simulink model "alt_dspbuilder_internal_ReadFIFO"  (Simulink 6.3)
settings: Solver=ode45  StartTime=0.0  StopTime=10.0  RelTol=1e-3
InitFcn:
  | %% DSPBuilder Start
  | alt_dspbuilder_update_model(bdroot)
  | %% DSPBuilder End
libraries: allblocks_alteradspbuilder2 x6
settings Model: Creator=cpurcell  LastModifiedBy=cpurcell
settings DebuggingCC: AlgebraicLoopMsg=none  MultiTaskCondExecSysMsg=none  StrictBusMsg=Warning
settings RTWCC: IncludeERTFirstTime=on
settings CodeAppCC: CustomSymbolStrType=$N$R$M

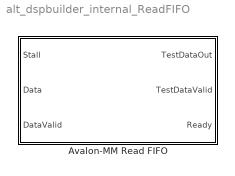
== system alt_dspbuilder_internal_ReadFIFO ==
  Avalon-MM Read FIFO : Subsystem  mask(Avalon-MM Read FIFO AlteraBlockSet){sgn=Signed Integer, bwl=8, bwr=3, depth=11, burst=0}
      mask prompts: sgn "Data Type"; bwl "[number of bits].[]"; bwr "[].[number of bits]"; depth "FIFO Depth"; burst "Max Burst"
      mask help:
      | Avalon-MM Read FIFO
      |
      | Implements a FIFO with Avalon-MM connectivity. Accessed by other Avalon-MM peripherals to obtain datawhen connected in SOPC Builder.
      |
      | Inputs:
      | Stall - Connect to Simulink blocks.
      | 	Used to simulate stall conditions of the Avalon-MM bus.
      | Data - Connect to DSP Builder blocks.
      | 	Used to collect outgoing data from the user design.
      | DataValid - Connect to DSP Builder blocks.
      | 	Should be asserted whenever the signal on the Data port corresponds to real data.
      |
      | Outputs:
      | TestDataOut - Connect to Simulink blocks.
      | 	Corresponds to the data received over the Avalon-MM bus.
      | TestDataValid - Connect to Simulink blocks.
      | 	Asserted whenever TestDataOut corresponds to real data.
      | Ready	- Connect to DSP Builder blocks.
      | 	Used to indicate that the block is ready to receive data.
      mask init:
      | alt_dspbuilder_internal_AvalonFIFO_Init(gcb,1,1, bwl,bwr,depth,burst);
      settings: CopyFcn=set_param(gcbh,'LinkStatus','none');
      mask Help: helpview(fullfile(alt_dspbuilder_get_quartus_rootdir, 'dsp_builder', 'docs', 'AvalonReadFIFO.html'))
      mask StyleString: popup(Signed Integer|Signed Fractional|Unsigned Integer),edit,edit,edit,edit
      mask CallbackString: alt_dspbuilder_internal_AvalonFIFO_Init(gcb,1,0);||||

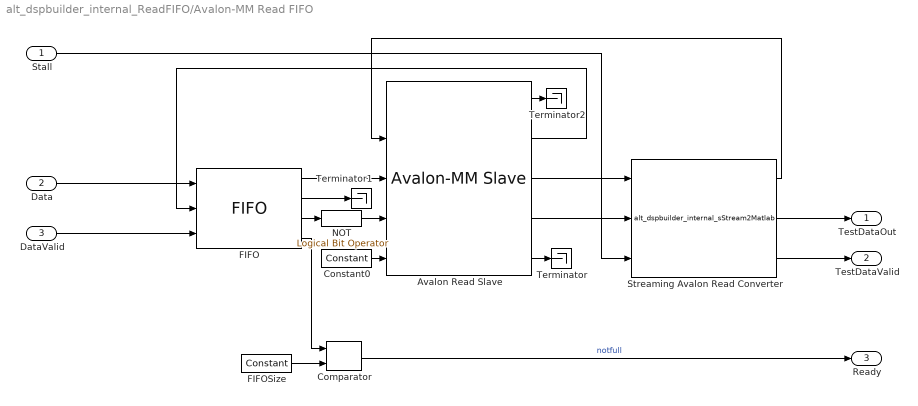
== system alt_dspbuilder_internal_ReadFIFO/Avalon-MM Read FIFO ==
  Stall : Inport
  Data : Inport  Port=2
  DataValid : Inport  Port=3
  Avalon Read Slave : allblocks_alteradspbuilder2/Avalon-MM Slave  iofile=C:\DOCUME~1\cpurcell\LOCALS~1\Temp\tb_tp293677\tp293677_Avalon-MM+Read+FIFO_Avalon+Read+Slave_address.salt,C:\DOCUME~1\cpurcell\LOCALS~1\Temp\tb_tp293677\tp293677_Avalon-MM+Read+FIFO_Avalon+Read+Slave_read.salt,C:\DOCUME~1\cpurcell\LOCALS~1\Temp\tb_tp293677\tp293677_Avalon-MM+Read+FIFO_Avalon+Read+Slave_readdata.capture,C:\DOCUME~1\cpurcell\LOCALS~1\Temp\tb_tp293677\tp293677_Avalon-MM+Read+FIFO_Avalon+Read+Slave_dataavailable.capture,C:\DOCUME~1\cpurcell\LOCALS~1\Temp\tb_tp293677\tp293677_Avalon-MM+Read+FIFO_Avalon+Read+Slave_endofpacket.capture,  SpecifyClock=off  clock=clock  addrWidth=2  addrAlignment=Dynamic  addrType=Read  BusType=Signed Integer  bwl=bwl  bwr=bwr  byteEnable=off  flowCtrl=on  pipeline=off  waitStateFormat=Fixed  readWaitStateCycles=0  writeWaitStateCycles=0  readLatencyFormat=Fixed  readLatencyCycles=0  burst=off  maxBurst=burst  irq=off  receiveBeginTransfer=off  useChipSelect=off  PORTTYPE=Output
  Comparator : allblocks_alteradspbuilder2/Comparator  direction=a < b
  Constant0 : allblocks_alteradspbuilder2/Constant  mask_cst=0  BusType=Single Bit  bwl=1  bwr=0  SpecifyClock=off
  FIFO : allblocks_alteradspbuilder2/FIFO  numwords=depth  BusType=Signed Integer  bwl=bwl  bwr=bwr  ram_type=AUTO  use_sclr=off  use_les_only=off  showahead_mode=off
  FIFOSize : allblocks_alteradspbuilder2/Constant  mask_cst=depth - 2  BusType=Unsigned Integer  bwl=ceil(log2(depth -1))  bwr=0  SpecifyClock=off
  NOT : allblocks_alteradspbuilder2/Logical Bit Operator  LogicalOperator=NOT  user_inputs=2
  Streaming Avalon Read Converter : S-Function  FunctionName=alt_dspbuilder_internal_sStream2Matlab  Parameters=-1
      mask Display:
      | port_label('input', 1, 'ReadData');
      | port_label('input', 2, 'DataAvailable');
      | port_label('input', 3, 'Stall');
      | port_label('output', 1, 'Read');
      | port_label('output', 2, 'TestData');
      | port_label('output', 3, 'TestDataValid');
  Terminator : Terminator
  Terminator1 : Terminator
  Terminator2 : Terminator
  TestDataOut : Outport
  TestDataValid : Outport  Port=2
  Ready : Outport  Port=3
  wires:
  DataValid/1 -> FIFO/3
  FIFO/3 -> NOT/1
  NOT/1 -> Avalon Read Slave/4
  Data/1 -> FIFO/1
  FIFO/1 -> Avalon Read Slave/3
  Avalon Read Slave/2 -> FIFO/2
  Streaming Avalon Read Converter/2 -> TestDataOut/1
  Streaming Avalon Read Converter/3 -> TestDataValid/1
  Streaming Avalon Read Converter/1 -> Avalon Read Slave/2
  Avalon Read Slave/3 -> Streaming Avalon Read Converter/1
  Constant0/1 -> Avalon Read Slave/5
  FIFO/4 -> Comparator/1
  Comparator/1 -> Ready/1  "notfull"
  Stall/1 -> Streaming Avalon Read Converter/3
  Avalon Read Slave/4 -> Streaming Avalon Read Converter/2
  Avalon Read Slave/5 -> Terminator/1
  FIFOSize/1 -> Comparator/2
  FIFO/2 -> Terminator1/1
  Avalon Read Slave/1 -> Terminator2/1
